simulink model "quadcopter_ekdf_test"  (R2015b)
settings: Solver=VariableStepAuto  StartTime=0.0  StopTime=50  RelTol=1e-3
values from neighbouring files (symbols this model uses):
  EKDF_K0 = 1    [init_ekdf_test.m]
  EKDF_P0 = 1    [init_ekdf_test.m]
  EKDF_Q = 1    [init_ekdf_test.m]
  EKDF_R = 1    [init_ekdf_test.m]
undefined symbols (not defined in the file or in its folder): Do, euleranglelim, Io, N, omegalim, Po, seed
libraries: vrlib x2, simulink x2
settings Model: Creator=Daniel  LastModifiedBy=mgreiff
settings SolverCC: AlgebraicLoopSolver=LineSearch

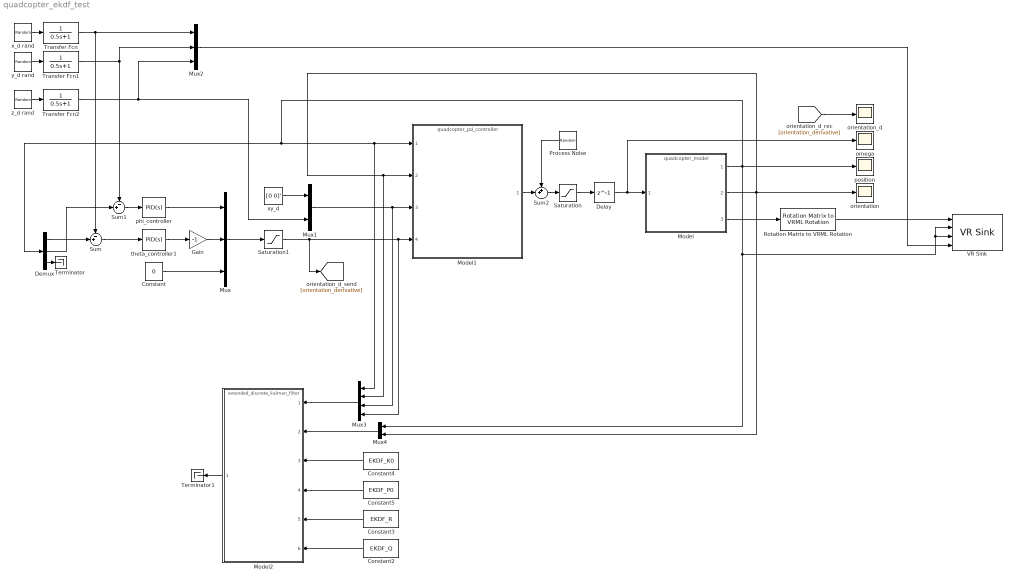
== system quadcopter_ekdf_test ==
  Constant : Constant  Value=0
  Constant2 : Constant  Value=EKDF_Q
  Constant3 : Constant  Value=EKDF_R
  Constant4 : Constant  Value=EKDF_K0
  Constant5 : Constant  Value=EKDF_P0
  Delay : Delay  DelayLength=1  InitialCondition=0  SampleTime=0.01
  Demux : Demux  Outputs=3
  Gain : Gain  Gain=-1
  Model : ModelReference  ModelNameDialog=quadcopter_model.mdl  SimulationMode=Normal  ModelReferenceVersion=1.114  CopyOfModelName=quadcopter_model.mdl
  Model1 : ModelReference  ModelNameDialog=quadcopter_pd_controller.mdl  SimulationMode=Normal  ModelReferenceVersion=1.59  CopyOfModelName=quadcopter_pd_controller.mdl
  Model2 : ModelReference  ModelNameDialog=extended_discrete_kalman_filter.slx  SimulationMode=Normal  ModelReferenceVersion=1.1  CopyOfModelName=extended_discrete_kalman_filter.slx
  Mux : Mux  Inputs=3
  Mux1 : Mux  Inputs=2
  Mux2 : Mux  Inputs=3
  Mux3 : Mux
  Mux4 : Mux  Inputs=2
  Process Noise : RandomNumber  Mean=[0 0 0 0]'  Variance=150  SampleTime=0.5
  Rotation Matrix to VRML Rotation : vrlib/Utilities/Rotation Matrix to VRML Rotation  maxzero=1e-12
  Saturation : Saturate  UpperLimit=omegalim(2)  LowerLimit=omegalim(1)
  Saturation1 : Saturate  UpperLimit=euleranglelim(2)  LowerLimit=euleranglelim(1)
  Sum : Sum  Inputs=-+|
  Sum1 : Sum  Inputs=-+|
  Sum2 : Sum  Inputs=++|
  Terminator : Terminator
  Terminator1 : Terminator
  Transfer Fcn : TransferFcn  Denominator=[0.5 1]
  Transfer Fcn1 : TransferFcn  Denominator=[0.5 1]
  Transfer Fcn2 : TransferFcn  Denominator=[0.5 1]
  VR Sink : vrlib/VR Sink  InstantiateOnLoad=on  SampleTime=0.05  ViewEnable=on  RemoteChange=off  RemoteView=off  FieldsWritten=copter.rotation.4.1.1.double#copter.translation.3.1.1.double#vp.translation.3.1.1.double#target.translation.3.1.1.double  WorldFileName=copter_world.wrl  WorldDescription=quadcopter_world  AutoView=on  VideoDimensions=[]  AllowVariableSize=off
  "omega " : Scope
  orientation : Scope
  orientation_d : Scope
  phi_controller : simulink/Continuous/PID Controller  Controller=PID  TimeDomain=Continuous-time  SampleTime=-1  IntegratorMethod=Forward Euler  FilterMethod=Forward Euler  Form=Parallel  UseFilter=on  ControllerParametersSource=internal  P=Po  I=Io  D=Do  N=N  InitialConditionSource=internal  InitialConditionForIntegrator=0  InitialConditionForFilter=0  ExternalReset=none  LimitOutput=off  UpperSaturationLimit=inf  LowerSaturationLimit=-inf  LinearizeAsGain=on  AntiWindupMode=none  Kb=1  TrackingMode=off  Kt=1  PParamMin=[]  PParamMax=[]  IParamMin=[]  IParamMax=[]  DParamMin=[]  DParamMax=[]  NParamMin=[]  NParamMax=[]  KbParamMin=[]  KbParamMax=[]  KtParamMin=[]  KtParamMax=[]  POutMin=[]  POutMax=[]  IOutMin=[]  IOutMax=[]  DOutMin=[]  DOutMax=[]  NOutMin=[]  NOutMax=[]  KbOutMin=[]  KbOutMax=[]  KtOutMin=[]  KtOutMax=[]  IntegratorOutMin=[]  IntegratorOutMax=[]  FilterOutMin=[]  FilterOutMax=[]  SumOutMin=[]  SumOutMax=[]  SumI1OutMin=[]  SumI1OutMax=[]  SumI2OutMin=[]  SumI2OutMax=[]  SumI3OutMin=[]  SumI3OutMax=[]  SumDOutMin=[]  SumDOutMax=[]  SaturationOutMin=[]  SaturationOutMax=[]  IntegratorContinuousStateAttributes=''  IntegratorStateMustResolveToSignalObject=off  IntegratorRTWStateStorageClass=Auto  FilterContinuousStateAttributes=''  FilterStateMustResolveToSignalObject=off  FilterRTWStateStorageClass=Auto  DifferentiatorICPrevScaledInput=0  DifferentiatorOutMin=[]  DifferentiatorOutMax=[]
  position : Scope
  theta_controller1 : simulink/Continuous/PID Controller  Controller=PID  TimeDomain=Continuous-time  SampleTime=-1  IntegratorMethod=Forward Euler  FilterMethod=Forward Euler  Form=Parallel  UseFilter=on  ControllerParametersSource=internal  P=Po  I=Io  D=Do  N=N  InitialConditionSource=internal  InitialConditionForIntegrator=0  InitialConditionForFilter=0  ExternalReset=none  LimitOutput=off  UpperSaturationLimit=inf  LowerSaturationLimit=-inf  LinearizeAsGain=on  AntiWindupMode=none  Kb=1  TrackingMode=off  Kt=1  PParamMin=[]  PParamMax=[]  IParamMin=[]  IParamMax=[]  DParamMin=[]  DParamMax=[]  NParamMin=[]  NParamMax=[]  KbParamMin=[]  KbParamMax=[]  KtParamMin=[]  KtParamMax=[]  POutMin=[]  POutMax=[]  IOutMin=[]  IOutMax=[]  DOutMin=[]  DOutMax=[]  NOutMin=[]  NOutMax=[]  KbOutMin=[]  KbOutMax=[]  KtOutMin=[]  KtOutMax=[]  IntegratorOutMin=[]  IntegratorOutMax=[]  FilterOutMin=[]  FilterOutMax=[]  SumOutMin=[]  SumOutMax=[]  SumI1OutMin=[]  SumI1OutMax=[]  SumI2OutMin=[]  SumI2OutMax=[]  SumI3OutMin=[]  SumI3OutMax=[]  SumDOutMin=[]  SumDOutMax=[]  SaturationOutMin=[]  SaturationOutMax=[]  IntegratorContinuousStateAttributes=''  IntegratorStateMustResolveToSignalObject=off  IntegratorRTWStateStorageClass=Auto  FilterContinuousStateAttributes=''  FilterStateMustResolveToSignalObject=off  FilterRTWStateStorageClass=Auto  DifferentiatorICPrevScaledInput=0  DifferentiatorOutMin=[]  DifferentiatorOutMax=[]
  x_d rand : UniformRandomNumber  Minimum=-30  Maximum=30  Seed=0+seed  SampleTime=10
  xy_d : Constant  Value=[0 0]'
  y_d rand : UniformRandomNumber  Minimum=-30  Maximum=30  Seed=1+seed  SampleTime=10
  z_d rand : UniformRandomNumber  Minimum=0  Maximum=15  Seed=2+seed  SampleTime=10
  wires:
  Model/2 -> Mux4/2, Mux3/2, Model1/2, orientation/1
  Model/1 -> Mux3/1, Model1/1, Demux/1, Mux4/1, VR Sink/2, VR Sink/3, position/1
  Saturation/1 -> Delay/1
  Model/3 -> Rotation Matrix to VRML Rotation/1
  Constant/1 -> Mux/3
  theta_controller1/1 -> Gain/1
  phi_controller/1 -> Mux/1
  Demux/3 -> Terminator/1
  Sum/1 -> theta_controller1/1
  Sum1/1 -> phi_controller/1
  x_d rand/1 -> Transfer Fcn/1
  y_d rand/1 -> Transfer Fcn1/1
  Gain/1 -> Mux/2
  Mux/1 -> Saturation1/1
  Demux/2 -> Sum1/2
  Demux/1 -> Sum/2
  Saturation1/1 -> [orientation_derivative], Mux3/4, Model1/4
  Mux1/1 -> Mux3/3, Model1/3
  xy_d/1 -> Mux1/1
  z_d rand/1 -> Transfer Fcn2/1
  Rotation Matrix to VRML Rotation/1 -> VR Sink/1
  Mux2/1 -> VR Sink/4
  Transfer Fcn/1 -> Mux2/1, Sum/1
  Transfer Fcn1/1 -> Sum1/1, Mux2/2
  Transfer Fcn2/1 -> Mux2/3, Mux1/2
  Process Noise/1 -> Sum2/1
  Sum2/1 -> Saturation/1
  Delay/1 -> "omega "/1, Model/1
  [orientation_derivative] -> orientation_d/1
  Model1/1 -> Sum2/2
  Constant2/1 -> Model2/6
  Constant3/1 -> Model2/5
  Mux3/1 -> Model2/1
  Mux4/1 -> Model2/2
  Model2/1 -> Terminator1/1
  Constant4/1 -> Model2/3
  Constant5/1 -> Model2/4
